simulink model "mdlref_counter_bus"  (Simulink 6.3)
settings: Solver=FixedStepDiscrete  StartTime=0.0  StopTime=10.0  FixedStep=Auto  RelTol=1e-3
PreLoadFcn:
  | load mdlref_counter_bus.mat
settings Model: Creator=The MathWorks Inc.  LastModifiedBy=batserve  ExtModeEnableOpenProtocolUploading=on  ExtModeOpenProtocolUploadingEqualLengthVectors=off  ExtModeAutoUpdateStatusClock=off  StrictBusMsg=ErrorLevel1
settings DataIOCC: SaveFormat=StructureWithTime  SignalLoggingName=logsOut
settings OptimizationCC: InlineParams=on  InlineInvariantSignals=on  BufferReusableBoundary=off
settings DebuggingCC: CheckExecutionContextPreStartOutputMsg=on  CheckExecutionContextRuntimeOutputMsg=on  SigSpecEnsureSampleTime=on  SignalResolutionControl=UseLocalSettings  SolverPrmCheckMsg=none
settings HardwareCC: TargetHWDeviceType=32-bit Generic
settings ModelReferenceCC: UpdateModelReferenceTargets=IfOutOfDate  CheckModelReferenceTargetMessage=none
settings RTWCC: GenerateReport=on  ProcessScript=grt_make_rtw_hook  LaunchReport=on

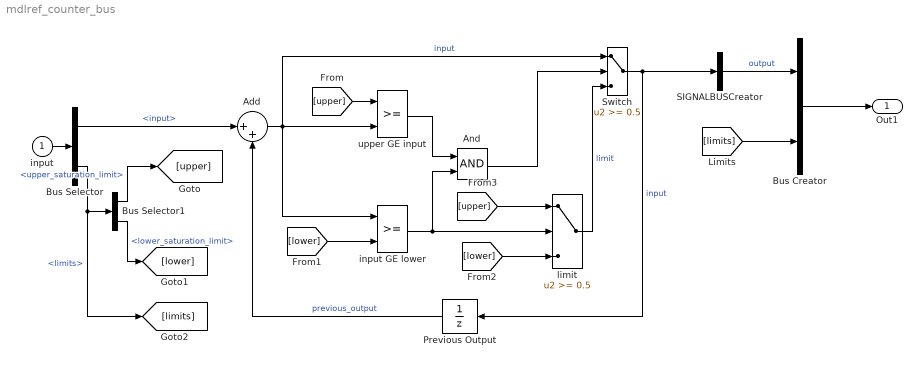
== system mdlref_counter_bus ==
  " input" : Inport  Port=1  UseBusObject=on
      settings: BusObject=COUNTERBUS
  " input GE lower" : RelationalOperator  Priority=1  InputSameDT=on
      settings: AttributesFormatString=\n
  " limit" : Switch  Threshold=0.5  SaturateOnIntegerOverflow=on  InputSameDT=on
  Add : Sum  Inputs=|++  OutScaling=2^-10
  And : Logic
  Bus Creator : BusCreator  Inputs='output','limits'  UseBusObject=on
      settings: BusObject=COUNTERBUS
  Bus Selector : BusSelector  OutputSignals=inputsignal.input,limits
  Bus Selector1 : BusSelector  OutputSignals=upper_saturation_limit,lower_saturation_limit
  Previous Output : UnitDelay  Orientation=left  SampleTime=-1
  SIGNALBUSCreator : BusCreator  Inputs=1  UseBusObject=on
      settings: BusObject=SIGNALBUS
  Switch : Switch  Threshold=0.5  SaturateOnIntegerOverflow=on  InputSameDT=on
  upper GE input : RelationalOperator  Priority=0  InputSameDT=on
      settings: AttributesFormatString=\n
  Out1 : Outport  UseBusObject=on
      settings: BusObject=COUNTERBUS
  wires:
  [upper] -> " limit"/1
  Switch/1 -> Previous Output/1, SIGNALBUSCreator/1  "input"
  " limit"/1 -> Switch/3  "limit"
  upper GE input/1 -> And/1
  Previous Output/1 -> Add/2  "previous_output"
  [lower] -> " limit"/3
  [upper] -> upper GE input/1
  [lower] -> " input GE lower"/2
  " input GE lower"/1 -> And/2, " limit"/2
  And/1 -> Switch/2
  Add/1 -> " input GE lower"/1, upper GE input/2, Switch/1  "input"
  " input"/1 -> Bus Selector/1
  Bus Selector/2 -> Bus Selector1/1, [limits]  "<limits>"
  Bus Selector/1 -> Add/1  "<input>"
  Bus Selector1/1 -> [upper]  "<upper_saturation_limit>"
  Bus Selector1/2 -> [lower]  "<lower_saturation_limit>"
  Bus Creator/1 -> Out1/1
  [limits] -> Bus Creator/2
  SIGNALBUSCreator/1 -> Bus Creator/1  "output"
